simulink model "B52SNSTest"  (R2023a)
settings: Solver=VariableStepAuto  StartTime=0.0  StopTime=100  RelTol=1E-4  AbsTol=1E-4
values from neighbouring files (symbols this model uses):
  AinfNarb_h_B52 = -61    [B52.m]    (also in CtrlParaSNSTuning.m)
  AinfNarb_p_B52 = 3    [B52.m]    (also in CtrlParaSNSTuning.m)
  AinfNarb_s_B52 = -1.0    (= -1)    [B52.m]    (also in CtrlParaSNSTuning.m)
  ANarb_B52_0 = 0.1    [B52.m]    (also in CtrlParaSNSTuning.m; InitPara.m)
  Cm_B52 = 0.01    [B52.m]    (also in CtrlParaSNSTuning.m)
  EL_B52 = -62    [B52.m]    (also in CtrlParaSNSTuning.m)
  ENarb_B52 = 30    [B52.m]    (also in CtrlParaSNSTuning.m)
  gL_B52 = 0.1    [B52.m]    (also in CtrlParaSNSTuning.m)
  gNarb_B52 = 0.1    [B52.m]    (also in CtrlParaSNSTuning.m)
  pNarb_B52 = 1    [B52.m]    (also in CtrlParaSNSTuning.m)
  RL_B52 = 0    [B52.m]    (also in CtrlParaSNSTuning.m)
  RNarb_B52 = 0    [B52.m]    (also in CtrlParaSNSTuning.m)
  tANarb_h_B52 = -60    [B52.m]    (also in CtrlParaSNSTuning.m)
  tANarb_p_B52 = 1.0    (= 1)    [B52.m]    (also in CtrlParaSNSTuning.m)
  tANarb_s_B52 = 5    [B52.m]    (also in CtrlParaSNSTuning.m)
  tANarb_tmax_B52 = 20    [B52.m]    (also in CtrlParaSNSTuning.m)
  tANarb_tmin_B52 = 5    [B52.m]    (also in CtrlParaSNSTuning.m)
  V_B52_0 = -60    [B52.m]    (also in CtrlParaSNSTuning.m = -62; InitPara.m = -62)
  V_max_B52 = (74.6788 - 0.0058) / 1.5 + 0.0058 + 1.95    (= 51.7378)    [CtrlParaSNSTuning.m]
  V_min_B52 = 0.0058 + 1.95    (= 1.9558)    [CtrlParaSNSTuning.m]
undefined symbols (not defined in the file or in its folder): Iapp, sigmarinf_B52, thetarinf_B52
settings Model: SimulationMode=accelerator  Creator=liyan  LastModifiedBy=Yanjun
settings ModelReferenceCC: EnableRefExpFcnMdlSchedulingChecks=on

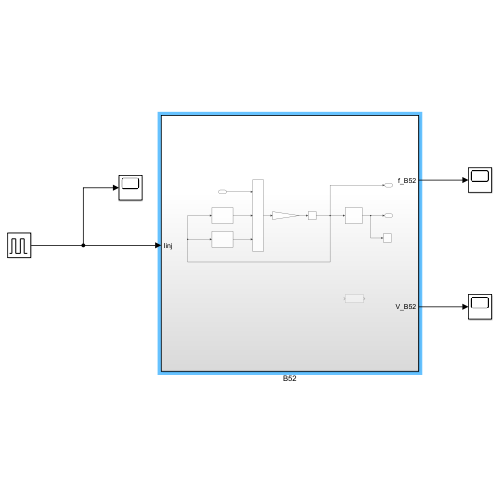
[thumbnail: Simulink's stored preview of the top-level diagram]
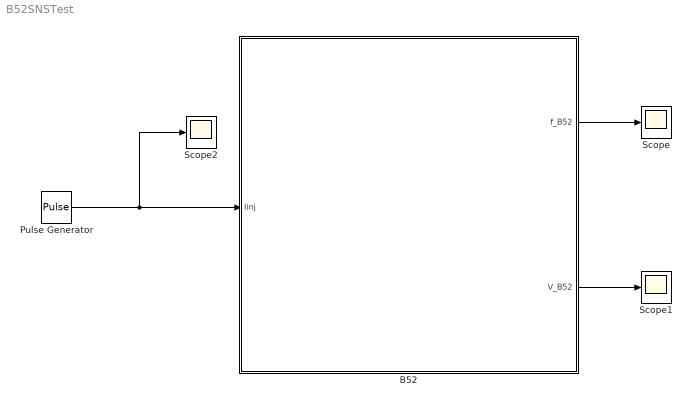
== system B52SNSTest ==
  B52 : Subsystem
  Pulse Generator : DiscretePulseGenerator  PulseType=Time based  Amplitude=Iapp  Period=100  PulseWidth=10/100*100  PhaseDelay=35
  Scope : Scope
  Scope1 : Scope
  Scope2 : Scope
  wires:
  Pulse Generator/1 -> B52/1(Iinj), Scope2/1
  B52/2(f_B52) -> Scope/1
  B52/1(V_B52) -> Scope1/1

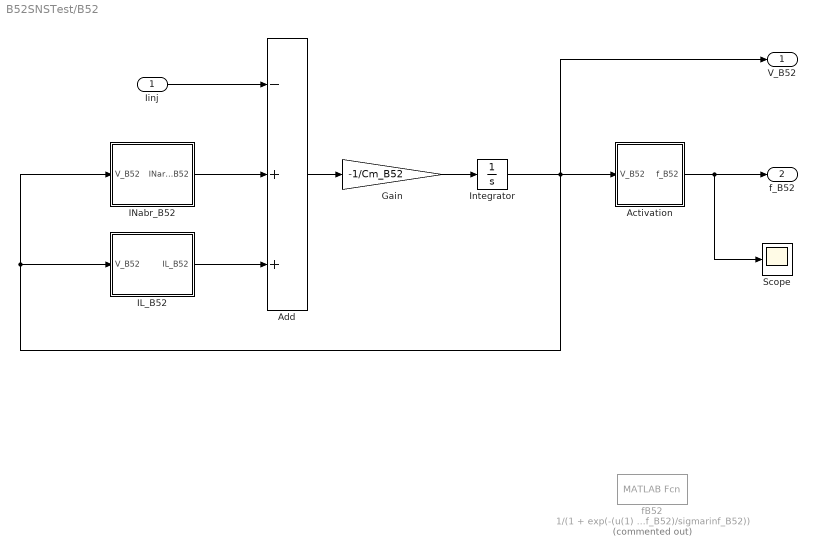
== system B52SNSTest/B52 ==
  Iinj : Inport
  Activation : Subsystem
  Add : Sum  Inputs=-++
  Gain : Gain  Gain=-1/Cm_B52
  IL_B52 : Subsystem
  INabr_B52 : Subsystem
  Integrator : Integrator  InitialCondition=V_B52_0
  Scope : Scope
  fB52 : MATLABFcn  Commented=on  MATLABFcn=1/(1 + exp(-(u(1) + thetarinf_B52)/sigmarinf_B52))
  V_B52 : Outport
  f_B52 : Outport  Port=2
  wires:
  Gain/1 -> Integrator/1
  Add/1 -> Gain/1
  IL_B52/1(IL_B52) -> Add/3
  Activation/1(f_B52) -> Scope/1, f_B52/1
  Integrator/1 -> Activation/1(V_B52), V_B52/1, IL_B52/1(V_B52), INabr_B52/1(V_B52)
  INabr_B52/1(INarb_B52) -> Add/2
  Iinj/1 -> Add/1

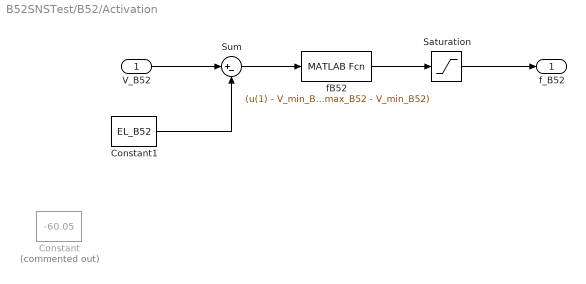
== system B52SNSTest/B52/Activation ==
  V_B52 : Inport
  Constant : Constant  Commented=on  Value=-60.05
  Constant1 : Constant  Value=EL_B52
  Saturation : Saturate  UpperLimit=1  LowerLimit=0
  Sum : Sum  Inputs=|+-
  fB52 : MATLABFcn  MATLABFcn=(u(1) - V_min_B52)/(V_max_B52 - V_min_B52)
  f_B52 : Outport
  wires:
  fB52/1 -> Saturation/1
  Saturation/1 -> f_B52/1
  Sum/1 -> fB52/1
  V_B52/1 -> Sum/1
  Constant1/1 -> Sum/2

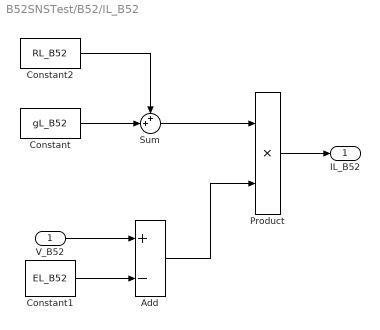
== system B52SNSTest/B52/IL_B52 ==
  V_B52 : Inport
  Add : Sum  Inputs=+-
  Constant : Constant  Value=gL_B52
  Constant1 : Constant  Value=EL_B52
  Constant2 : Constant  Value=RL_B52
  Product : Product
  Sum : Sum  Inputs=++|
  IL_B52 : Outport
  wires:
  Constant1/1 -> Add/2
  V_B52/1 -> Add/1
  Constant2/1 -> Sum/1
  Sum/1 -> Product/1
  Constant/1 -> Sum/2
  Add/1 -> Product/2
  Product/1 -> IL_B52/1

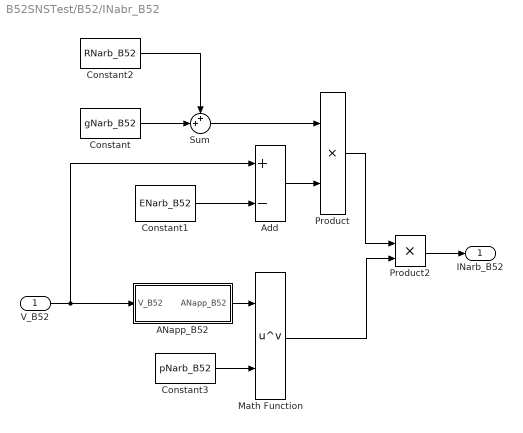
== system B52SNSTest/B52/INabr_B52 ==
  V_B52 : Inport
  ANapp_B52 : Subsystem
  Add : Sum  Inputs=+-
  Constant : Constant  Value=gNarb_B52
  Constant1 : Constant  Value=ENarb_B52
  Constant2 : Constant  Value=RNarb_B52
  Constant3 : Constant  Value=pNarb_B52
  Math Function : Math  Operator=pow
  Product : Product
  Product2 : Product
  Sum : Sum  Inputs=++|
  INarb_B52 : Outport
  wires:
  Add/1 -> Product/2
  Constant1/1 -> Add/2
  V_B52/1 -> ANapp_B52/1(V_B52), Add/1
  Product/1 -> Product2/1
  Math Function/1 -> Product2/2
  Product2/1 -> INarb_B52/1
  Constant/1 -> Sum/2
  Sum/1 -> Product/1
  Constant2/1 -> Sum/1
  ANapp_B52/1(ANapp_B52) -> Math Function/1
  Constant3/1 -> Math Function/2

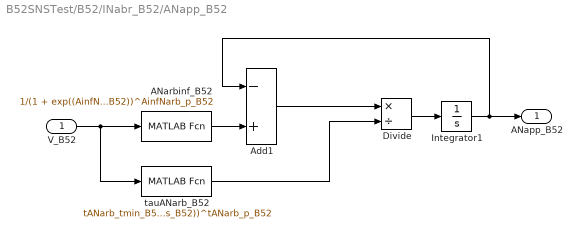
== system B52SNSTest/B52/INabr_B52/ANapp_B52 ==
  V_B52 : Inport
  ANarbinf_B52 : MATLABFcn  MATLABFcn=1/(1 + exp((AinfNarb_h_B52 - u(1))/AinfNarb_s_B52))^AinfNarb_p_B52
  Add1 : Sum  Inputs=-+
  Divide : Product  Inputs=*/
  Integrator1 : Integrator  InitialCondition=ANarb_B52_0
  tauANarb_B52 : MATLABFcn  MATLABFcn=tANarb_tmin_B52 + (tANarb_tmax_B52 - tANarb_tmin_B52)/(1 + exp((u(1) - tANarb_h_B52)/tANarb_s_B52))^tANarb_p_B52
  ANapp_B52 : Outport
  wires:
  tauANarb_B52/1 -> Divide/2
  Divide/1 -> Integrator1/1
  Integrator1/1 -> Add1/1, ANapp_B52/1
  Add1/1 -> Divide/1
  ANarbinf_B52/1 -> Add1/2
  V_B52/1 -> tauANarb_B52/1, ANarbinf_B52/1
